simulink model "signal_feedback_fop"  (R2024b)
settings: Solver=VariableStepAuto  StartTime=0.0  StopTime=100  RelTol=1e-3
undefined symbols (not defined in the file): C1, C2, G, R1, R2
libraries: spsSeriesRLCBranchLib x4, spsControlledVoltageSourceLib x2, spsVoltageMeasurementLib x2, simulink x1, spsGroundLib x1, sps_lib x1
settings Model: Creator=owner  LastModifiedBy=owner
settings DebuggingCC: AlgebraicLoopMsg=none

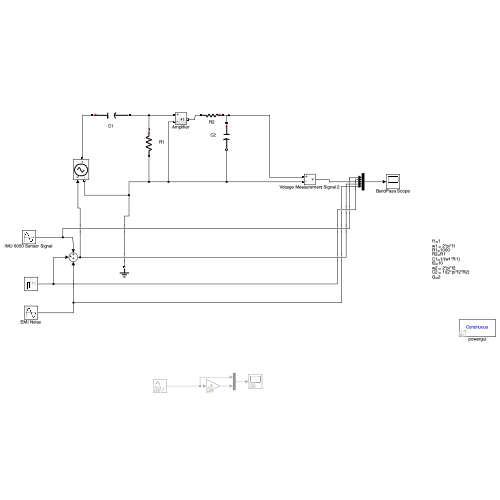
[thumbnail: Simulink's stored preview of the top-level diagram]
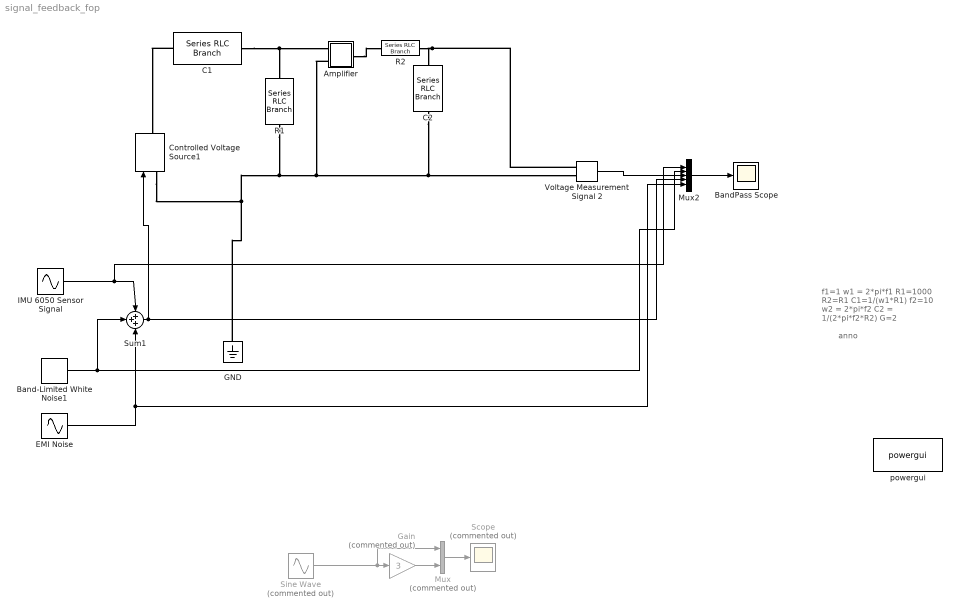
== system signal_feedback_fop ==
  note: f1=1
      | w1 = 2*pi*f1
      | R1=1000
      | R2=R1
      | C1=1/(w1*R1)
      | f2=10
      | w2 = 2*pi*f2
      | C2 = 1/(2*pi*f2*R2)
      | G=2
  note: anno
  Amplifier : Subsystem
  Band-Limited White Noise1 : simulink/Sources/Band-Limited White Noise  Cov=[0.1]  Ts=1  seed=[23341]
  BandPass Scope : Scope
  C1 : spsSeriesRLCBranchLib/Series RLC Branch  LConnTagsString=__new0  RConnTagsString=__new0  BranchType=C  Resistance=1  Inductance=1e-3  SetiL0=off  InitialCurrent=0  Capacitance=C1  Setx0=off  InitialVoltage=0  Measurements=None
  C2 : spsSeriesRLCBranchLib/Series RLC Branch  LConnTagsString=__new0  RConnTagsString=__new0  BranchType=C  Resistance=1  Inductance=1e-3  SetiL0=off  InitialCurrent=0  Capacitance=C2  Setx0=off  InitialVoltage=0  Measurements=None
  Controlled Voltage Source1 : spsControlledVoltageSourceLib/Controlled Voltage Source  Initialize=off  Source_Type=AC  Amplitude=0  Phase=0  Frequency=0  Measurements=Voltage
  EMI Noise : Sin  Amplitude=0.5  Frequency=324.1593  SampleTime=0
  GND : spsGroundLib/Ground  LConnTagsString=a
  Gain : Gain  Commented=on  Gain=3
  IMU 6050 Sensor Signal : Sin  Frequency=12.5664  SampleTime=0
  Mux : Mux  Commented=on  Inputs=2
  Mux2 : Mux  Inputs=5
  R1 : spsSeriesRLCBranchLib/Series RLC Branch  LConnTagsString=__new0  RConnTagsString=__new0  BranchType=R  Resistance=R1  Inductance=1e-3  SetiL0=off  InitialCurrent=0  Capacitance=1e-6  Setx0=off  InitialVoltage=0  Measurements=None
  R2 : spsSeriesRLCBranchLib/Series RLC Branch  LConnTagsString=__new0  RConnTagsString=__new0  BranchType=R  Resistance=R2  Inductance=1e-3  SetiL0=off  InitialCurrent=0  Capacitance=1e-6  Setx0=off  InitialVoltage=0  Measurements=None
  Scope : Scope  Commented=on
  Sine Wave : Sin  Commented=on  SampleTime=0
  Sum1 : Sum  Inputs=+++
  Voltage Measurement Signal 2 : spsVoltageMeasurementLib/Voltage Measurement  PhasorSimulation=off  OutputType=Complex  PSBequivalent=0
  powergui : sps_lib/powergui  Priority=1  SimulationMode=Continuous  SampleTime=50e-6  frequency=60  Iterations=50  frequencyindice=0  Pbase=100e6  ErrMax=1e-4  UnitsV=kV  UnitsW=MW  buscounter=0  FunctionMessages=off  echomessages=off  EnableUseOfTLC=off  CurrentSourceSwitches=off  DisableSnubberDevices=off  DisableRonSwitches=off  DisableVfSwitches=off  DisplayEquations=off  AutomaticDiscreteSolvers=off  SolverType=Tustin/Backward Euler (TBE)  Interpol=off  ExternalGateDelay=off  methode=off  Ts=100  x0status=blocks  SPID=on  SwTol=0  HookPort=off  NonlinearTolerance=1e-4  nMaxIteration=100  ContinueOnMaxIteration=off  RestoreLinks=warning  ResistiveCurrentMeasurement=off  Frange=[0:2:500]  Ylog=off  Xlog=on  ShowGrid=off  save=off  variable=ZData  structure=0  ZoomFFT=off  StartTime=0.0  cycles=1  DisplayStyle=1  fundamental=60  FreqAxis=off  MaxFrequency=1000  frequencyindicesteady=1  RmsSteady=1  display=off
  wires:
  Band-Limited White Noise1/1 -> Mux2/2, Sum1/2
  Sum1/1 -> Controlled Voltage Source1/1, Mux2/4
  EMI Noise/1 -> Sum1/3, Mux2/5
  Mux2/1 -> BandPass Scope/1
  IMU 6050 Sensor Signal/1 -> Mux2/1, Sum1/1
  Voltage Measurement Signal 2/1 -> Mux2/3
  Sine Wave/1 -> Mux/1, Gain/1
  Mux/1 -> Scope/1
  Gain/1 -> Mux/2
  connections:
  Voltage Measurement Signal 2/LConn1 -- R2/LConn1 -- C2/LConn1
  GND/LConn1 -- Controlled Voltage Source1/LConn1 -- Voltage Measurement Signal 2/LConn2 -- C2/RConn1 -- Amplifier/LConn2 -- R1/RConn1
  C1/LConn1 -- Controlled Voltage Source1/RConn1
  C1/RConn1 -- R1/LConn1 -- Amplifier/LConn1
  Amplifier/RConn1 -- R2/RConn1

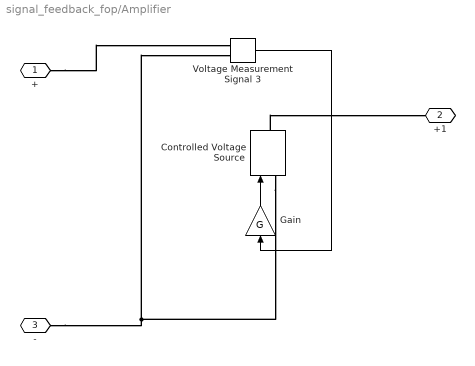
== system signal_feedback_fop/Amplifier ==
  Controlled Voltage Source : spsControlledVoltageSourceLib/Controlled Voltage Source  Initialize=on  Source_Type=AC  Amplitude=0  Phase=0  Frequency=0  Measurements=None
  Gain : Gain  Gain=G
  Voltage Measurement Signal 3 : spsVoltageMeasurementLib/Voltage Measurement  PhasorSimulation=off  OutputType=Complex  PSBequivalent=0
  + : PMIOPort  Side=Left
  +1 : PMIOPort  Port=2  Side=Right
  - : PMIOPort  Port=3  Side=Left
  wires:
  Voltage Measurement Signal 3/1 -> Gain/1
  Gain/1 -> Controlled Voltage Source/1
  connections:
  +/RConn1 -- Voltage Measurement Signal 3/LConn1
  Controlled Voltage Source/RConn1 -- +1/RConn1
  -/RConn1 -- Controlled Voltage Source/LConn1 -- Voltage Measurement Signal 3/LConn2
